simulink model "taller5"  (R2024b)
settings: Solver=FixedStepAuto  StartTime=0.0  StopTime=10.0  FixedStep=0.000001  RelTol=1e-3
settings Model: Creator=dvdmi  LastModifiedBy=dvdmi

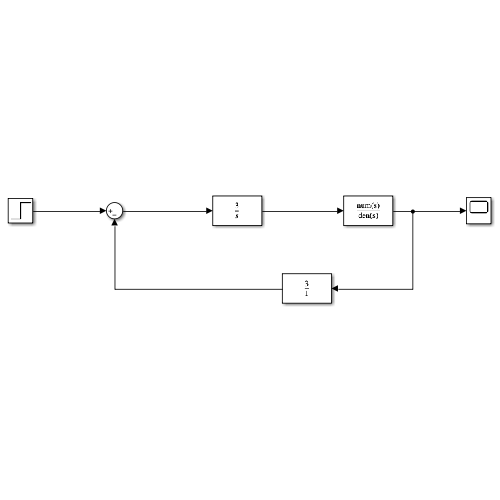
[thumbnail: Simulink's stored preview of the top-level diagram]
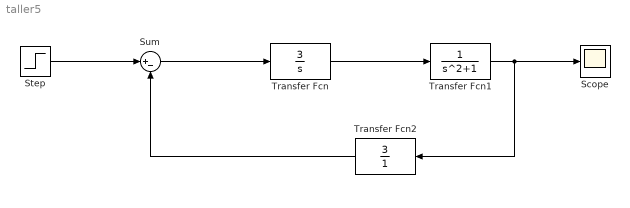
== system taller5 ==
  Scope : Scope
  Step : Step  SampleTime=0
  Sum : Sum  Inputs=|+-
  Transfer Fcn : TransferFcn  Numerator=[3]  Denominator=[1 0]
  Transfer Fcn1 : TransferFcn  Denominator=[1 0 1]
  Transfer Fcn2 : TransferFcn  Numerator=[3]  Denominator=[0 1]
  wires:
  Sum/1 -> Transfer Fcn/1
  Transfer Fcn/1 -> Transfer Fcn1/1
  Transfer Fcn1/1 -> Scope/1, Transfer Fcn2/1
  Transfer Fcn2/1 -> Sum/2
  Step/1 -> Sum/1
